simulink model "oscillator2"  (R2018b)
settings: Solver=FixedStepAuto  StartTime=0.0  StopTime=40  FixedStep=0.001  RelTol=1e-3
settings Model: Creator=User  LastModifiedBy=User

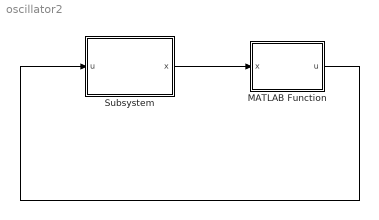
== system oscillator2 ==
  MATLAB Function : MATLAB Function  TreatAsAtomicUnit=on
  Subsystem : Subsystem
  wires:
  Subsystem/1(x) -> MATLAB Function/1(x)
  MATLAB Function/1(u) -> Subsystem/1(u)

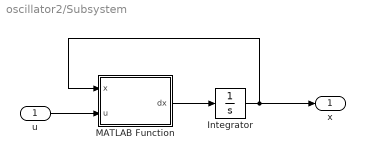
== system oscillator2/Subsystem ==
  u : Inport
  Integrator : Integrator  InitialCondition=[0;1]
  MATLAB Function : MATLAB Function  TreatAsAtomicUnit=on
  x : Outport
  wires:
  Integrator/1 -> x/1, MATLAB Function/1(x)
  MATLAB Function/1(dx) -> Integrator/1
  u/1 -> MATLAB Function/2(u)

== matlab function oscillator2/MATLAB Function ==
  data: x input; u output
function u = fcn(x)
x1=x(1);
x2=x(2);
u=-tanh(3.5738*x1+5.0619*x2-0.0646*x2^3-6.5706*x1^3-14.0109*x1^2*x2-12.2683*x1*x2^2-5.5855*x2^5+3.7739*x1^5+12.4929*x1^4*x2+19.9311*x1^3*x2^2+9.3338*x1^2*x2^3+5.6905*x1*x2^4+2.6474*x2^7-0.3696*x1^7-2.8634*x1^6*x2-7.7255*x1^5*x2^2-7.3681*x1^4*x2^3-6.2633*x1^3*x2^4+1.3101*x1^2*x2^5-0.1391*x1*x2^6);
end

== matlab function oscillator2/Subsystem/MATLAB Function ==
  data: x input; u input; dx output
function dx = fcn(x,u)
x1=x(1);
x2=x(2);
dx=[x1+x2-x1*(x1^2+x2^2);
    -x1+x2-x2*(x1^2+x2^2)+u];
end
